simulink model "Problem5"  (R2020b)
settings: Solver=VariableStepAuto  StartTime=0.0  StopTime=10.0  RelTol=1e-3
values from neighbouring files (symbols this model uses):
  C = 10e-6    (= 1e-05)    [Prob5.m]
  R = 10    [Prob5.m]
settings Model: Creator=Dell  LastModifiedBy=Dell

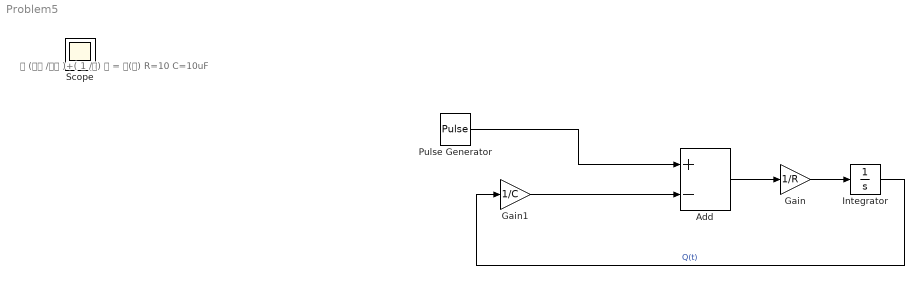
== system Problem5 ==
  note: 𝑅 (𝑑𝑄 /𝑑𝑡 )+( 1 /𝐶) 𝑄 = 𝐸(𝑡)
      | R=10
      | C=10uF
  Add : Sum  Inputs=+-
  Gain : Gain  Gain=1/R
  Gain1 : Gain  Gain=1/C
  Integrator : Integrator
  Pulse Generator : DiscretePulseGenerator  PulseType=Time based  Period=10  PulseWidth=5
  Scope : Scope
  wires:
  Add/1 -> Gain/1
  Gain/1 -> Integrator/1
  Integrator/1 -> Gain1/1  "Q(t)"
  Gain1/1 -> Add/2
  Pulse Generator/1 -> Add/1
